simulink model "ZIEGLER_NICHOLS"  (R2018b)
settings: Solver=VariableStepAuto  StartTime=0.0  StopTime=15  RelTol=1e-3
libraries: simulink x6
settings Model: Creator=DELL  LastModifiedBy=DELL

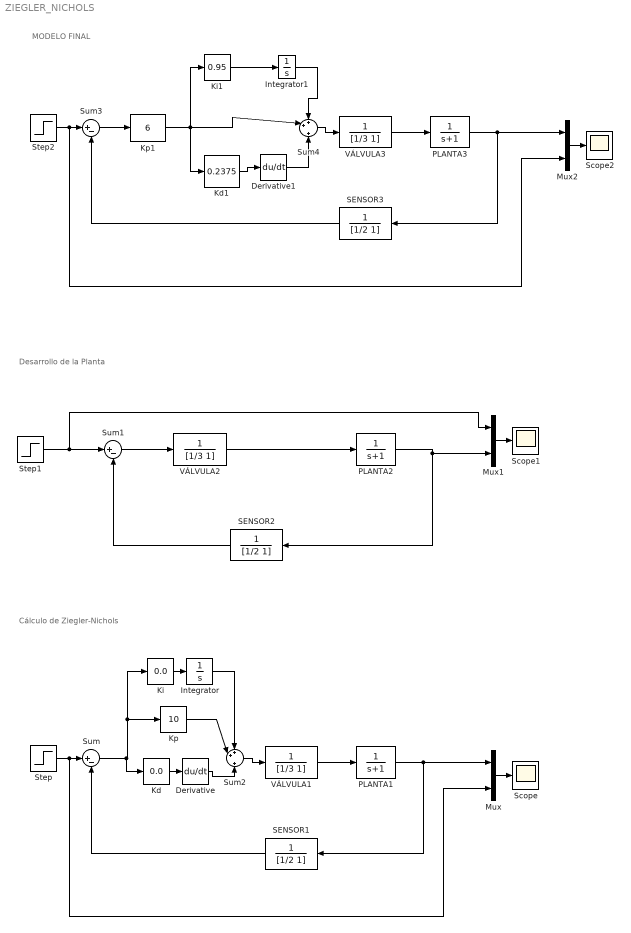
== system ZIEGLER_NICHOLS ==
  note: Cálculo de Ziegler-Nichols
  note: Desarrollo de la Planta
  note: MODELO FINAL
  Derivative : Derivative
  Derivative1 : Derivative
  Integrator : Integrator
  Integrator1 : Integrator
  Kd : simulink/Math Operations/Slider Gain  gain=0.0  low=0  high=20
  Kd1 : simulink/Math Operations/Slider Gain  gain=0.2375  low=0  high=20
  Ki : simulink/Math Operations/Slider Gain  gain=0.0  low=0  high=20
  Ki1 : simulink/Math Operations/Slider Gain  gain=0.95  low=0  high=20
  Kp : simulink/Math Operations/Slider Gain  gain=10  low=0  high=20
  Kp1 : simulink/Math Operations/Slider Gain  gain=6  low=0  high=20
  Mux : Mux  Inputs=2
  Mux1 : Mux  Inputs=2
  Mux2 : Mux  Inputs=2
  PLANTA1 : TransferFcn  Denominator=[1 1]
  PLANTA2 : TransferFcn  Denominator=[1 1]
  PLANTA3 : TransferFcn  Denominator=[1 1]
  SENSOR1 : TransferFcn  Denominator=[1/2 1]
  SENSOR2 : TransferFcn  Denominator=[1/2 1]
  SENSOR3 : TransferFcn  Denominator=[1/2 1]
  Scope : Scope
  Scope1 : Scope
  Scope2 : Scope
  Step : Step  SampleTime=0
  Step1 : Step  Time=0  SampleTime=0
  Step2 : Step  SampleTime=0
  Sum : Sum  Inputs=|+-
  Sum1 : Sum  Inputs=|+-
  Sum2 : Sum  Inputs=++|+
  Sum3 : Sum  Inputs=|+-
  Sum4 : Sum  Inputs=++|+
  VÁLVULA1 : TransferFcn  Denominator=[1/3 1]
  VÁLVULA2 : TransferFcn  Denominator=[1/3 1]
  VÁLVULA3 : TransferFcn  Denominator=[1/3 1]
  wires:
  Integrator/1 -> Sum2/1
  Mux/1 -> Scope/1
  Derivative/1 -> Sum2/3
  Ki/1 -> Integrator/1
  Kp/1 -> Sum2/2
  Kd/1 -> Derivative/1
  Sum/1 -> Kd/1, Ki/1, Kp/1
  PLANTA1/1 -> SENSOR1/1, Mux/1
  VÁLVULA1/1 -> PLANTA1/1
  SENSOR1/1 -> Sum/2
  Sum2/1 -> VÁLVULA1/1
  Step/1 -> Mux/2, Sum/1
  PLANTA2/1 -> Mux1/2, SENSOR2/1
  Step1/1 -> Mux1/1, Sum1/1
  SENSOR2/1 -> Sum1/2
  Mux1/1 -> Scope1/1
  VÁLVULA2/1 -> PLANTA2/1
  Sum1/1 -> VÁLVULA2/1
  Ki1/1 -> Integrator1/1
  Integrator1/1 -> Sum4/1
  Kd1/1 -> Derivative1/1
  Sum4/1 -> VÁLVULA3/1
  PLANTA3/1 -> SENSOR3/1, Mux2/1
  Step2/1 -> Mux2/2, Sum3/1
  SENSOR3/1 -> Sum3/2
  Mux2/1 -> Scope2/1
  VÁLVULA3/1 -> PLANTA3/1
  Derivative1/1 -> Sum4/3
  Sum3/1 -> Kp1/1
  Kp1/1 -> Kd1/1, Ki1/1, Sum4/2
